simulink model "frequence_response_integrators"  (R2019b)
settings: Solver=ode45  StartTime=0.0  StopTime=80  RelTol=1e-3  EnableMultiTasking=on
values from neighbouring files (symbols this model uses):
  A1 = 4    [es1.m]
  A2 = 6    [es1.m]
  C = [1 1 0 0;0 0 1 1]    [es1.m]
  t1 = 2    [es1.m]
  t2 = 10    [es1.m]
undefined symbols (not defined in the file or in its folder): A, B, D
settings Model: Creator=stefano  LastModifiedBy=Chiara
settings DataIOCC: LimitDataPoints=on  SaveFormat=Array  SignalLoggingSaveFormat=ModelDataLogs  ReturnWorkspaceOutputs=off
settings OptimizationCC: ExpressionDepthLimit=2147483647  LifeSpan=inf
settings DebuggingCC: UnderspecifiedInitializationDetection=Classic  MergeDetectMultiDrivingBlocksExec=none  SolverPrmCheckMsg=warning  FcnCallInpInsideContextMsg=warning  StateNameClashWarn=warning  SFUnexpectedBacktrackingDiag=warning  SFNoUnconditionalDefaultTransitionDiag=warning  SFExecutionAtInitializationDiag=none  ArithmeticOperatorsInVariantConditions=warning
settings HardwareCC: ProdBitPerPointer=32  ProdBitPerSizeT=32  ProdBitPerPtrDiffT=32  ProdLargestAtomicFloat=None  ProdIntDivRoundTo=Undefined  ProdEndianess=Unspecified  ProdWordSize=32  ProdHWDeviceType=32-bit Generic
settings ModelReferenceCC: PropagateSignalLabelsOutOfModel=off
settings SFSimCC: SimUseLocalCustomCode=off  CustomCodeUndefinedFunction=UseInterfaceOnly
settings RTWCC: RTWUseLocalCustomCode=off
settings CodeAppCC: StateflowObjectComments=on
settings GRTTargetCC: TargetLangStandard=C89/C90 (ANSI)  GeneratePreprocessorConditionals=Disable all  CombineOutputUpdateFcns=off  GRTInterface=on
settings ConfigComp: CovMetricSettings=dw  CovHtmlReporting=on  CovSaveCumulativeToWorkspaceVar=on  CovSaveSingleToWorkspaceVar=on  CovExternalEMLEnable=off

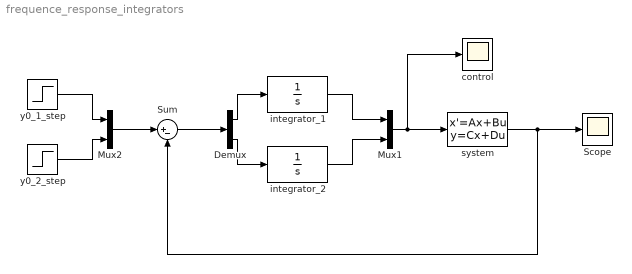
== system frequence_response_integrators ==
  Demux : Demux  Outputs=2
  Mux1 : Mux  Inputs=2
  Mux2 : Mux  Inputs=2
  Scope : Scope
  Sum : Sum  Inputs=|+-
  control : Scope
  integrator_1 : TransferFcn  Denominator=[1 0]
  integrator_2 : TransferFcn  Denominator=[1 0]
  system : StateSpace  A=A  B=B  C=C  D=D  InitialCondition=0
  y0_1_step : Step  Time=t1  After=A1  SampleTime=0
  y0_2_step : Step  Time=t2  After=A2  SampleTime=0
  wires:
  system/1 -> Scope/1, Sum/2
  Mux2/1 -> Sum/1
  Sum/1 -> Demux/1
  Mux1/1 -> system/1, control/1
  integrator_1/1 -> Mux1/1
  Demux/1 -> integrator_1/1
  Demux/2 -> integrator_2/1
  integrator_2/1 -> Mux1/2
  y0_2_step/1 -> Mux2/2
  y0_1_step/1 -> Mux2/1
